simulink model "CANRXcommunicationunit_2"  (R2024a)
settings: Solver=VariableStepAuto  StartTime=0.0  StopTime=10.0  RelTol=1e-3
undefined symbols (not defined in the file or in its folder): canChannel
libraries: canlib x2, canmsglib x2
settings Model: DataDictionary=BMS_System_dict1.sldd  Creator=hirah  LastModifiedBy=hirah

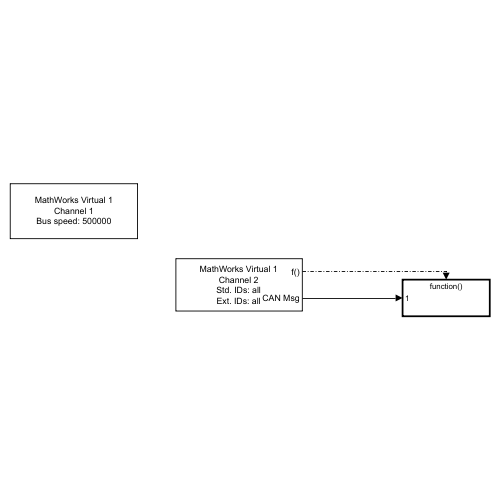
[thumbnail: Simulink's stored preview of the top-level diagram]
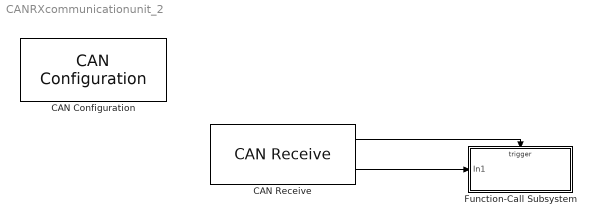
== system CANRXcommunicationunit_2 ==
  CAN Configuration : canlib/CAN Configuration  BlockHandle=570.0001  Device=MathWorks Virtual 1 (Channel 1)  DeviceMenu=MathWorks Virtual 1 (Channel 1)  ObjConstructor=canChannel('MathWorks', 'Virtual 1', 1)  BusSpeed=500000  EnableBitParameters=off  AckMode=Normal
  CAN Receive : canlib/CAN Receive  BlockHandle=729.0002  Device=MathWorks Virtual 1 (Channel 2)  DeviceMenu=MathWorks Virtual 1 (Channel 2)  ObjConstructor=canChannel('MathWorks', 'Virtual 1', 2)  EnableStandardIDsFilter=off  StdIDsCombo=Allow all  StandardIDs=261  EnableExtendedIDsFilter=off  ExtIDsCombo=Allow all  ExtendedIDs=0  SampleTime=0.01  MsgsPerTimestep=all  InternalFilterUpdateStatus=on  BusOutput=off
  Function-Call Subsystem : Subsystem  TreatAsAtomicUnit=on
  wires:
  CAN Receive/1 -> Function-Call Subsystem/Trigger
  CAN Receive/2 -> Function-Call Subsystem/1(In1)

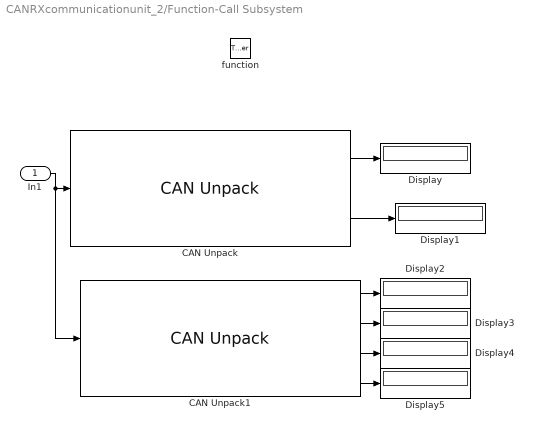
== system CANRXcommunicationunit_2/Function-Call Subsystem ==
  In1 : Inport
  function : TriggerPort  TriggerType=function-call  VariantControl=(inherit)
  CAN Unpack : canmsglib/CAN Unpack  CANdbFile=C:\Users\hirah\Downloads\BMS_CAN_Database (5).dbc  MsgList=frmBMStoVCU  MsgName=frmBMStoVCU  MsgIDType=Standard (11-bit identifier)  MsgIdentifier=321  MsgLength=2  SignalInfo={ 'sigBMSFaultStatus', '8', '8', 'LE', 'unsigned', 'Standard', '0', '1', '0', '0', '3'; 'sigBMSOperatingMode', '0', '8', 'LE', 'unsigned', 'Standard', '0', '1', '0', '0', '5' }  IDPort=off  TimestampPort=off  ErrorPort=off  RemotePort=off  LengthPort=off  StatusPort=off  ApplyMinMax=off
      settings: DataFormat=CANdb specified signals
  CAN Unpack1 : canmsglib/CAN Unpack  CANdbFile=C:\Users\hirah\Downloads\BMS_CAN_Database (5).dbc  MsgList=frmBMSStateEstimation  MsgName=frmBMSStateEstimation  MsgIDType=Standard (11-bit identifier)  MsgIdentifier=259  MsgLength=6  SignalInfo={ 'sigSOC', '0', '8', 'LE', 'unsigned', 'Standard', '0', '1', '0', '0', '100'; 'sigSOH', '8', '8', 'LE', 'unsigned', 'Standard', '0', '1', '0', '0', '100'; 'sigSOPCharge', '32', '16', 'LE', 'unsigned', 'Standard', '0', '1', '0', '0', '200'; 'sigSOPDischarge', '16', '16', 'LE', 'unsigned', 'Standard', '0', '1', '0', '0', '200' }  IDPort=off  TimestampPort=off  ErrorPort=off  RemotePort=off  LengthPort=off  StatusPort=off  ApplyMinMax=off
      settings: DataFormat=CANdb specified signals
  Display{,1..5} (6 alike) : Display
  wires:
  In1/1 -> CAN Unpack1/1, CAN Unpack/1
  CAN Unpack/1 -> Display/1
  CAN Unpack/2 -> Display1/1
  CAN Unpack1/4 -> Display5/1
  CAN Unpack1/3 -> Display4/1
  CAN Unpack1/2 -> Display3/1
  CAN Unpack1/1 -> Display2/1
